simulink model "Bicycle_Model"  (R2019b)
settings: Solver=ode45  StartTime=0.0  StopTime=10.0  MaxStep=0.2  RelTol=1e-3
libraries: simulink x2
settings Model: Creator=Liam  LastModifiedBy=yafta
settings DataIOCC: ReturnWorkspaceOutputs=off
settings DebuggingCC: ArithmeticOperatorsInVariantConditions=warning
settings SFSimCC: SimUseLocalCustomCode=off  CustomCodeUndefinedFunction=UseInterfaceOnly
settings RTWCC: RTWUseLocalCustomCode=off

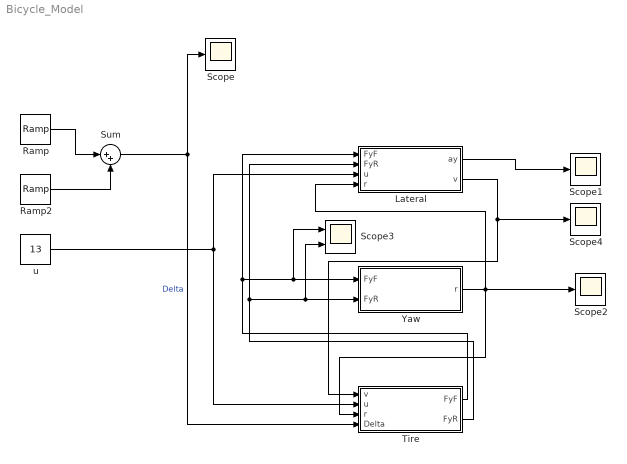
== system Bicycle_Model ==
  Lateral : Subsystem
  Ramp : simulink/Sources/Ramp  slope=0.05  start=1  InitialOutput=0
  Ramp2 : simulink/Sources/Ramp  slope=-0.05  start=5  InitialOutput=0
  Scope{,1..2,4} (4 alike) : Scope
  Scope3 : Scope  NumInputPorts=2
  Sum : Sum  Inputs=|++
  Tire : Subsystem
  Yaw : Subsystem
  u : Constant  Value=13
  wires:
  u/1 -> Tire/2(u), Lateral/3(u)
  Yaw/1(r) -> Lateral/4(r), Tire/3(r), Scope2/1
  Tire/1(FyF) -> Lateral/1(FyF), Scope3/1, Yaw/1("FyF ")
  Tire/2(FyR) -> Lateral/2(FyR), Scope3/2, Yaw/2(FyR)
  Ramp/1 -> Sum/1
  Ramp2/1 -> Sum/2
  Sum/1 -> Scope/1, Tire/4("Delta ")  "Delta"
  Lateral/1(ay) -> Scope1/1
  Lateral/2(v) -> Tire/1(v), Scope4/1

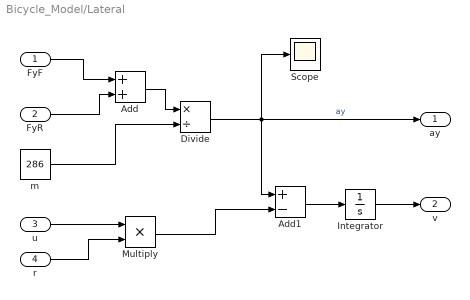
== system Bicycle_Model/Lateral ==
  FyF : Inport
  FyR : Inport  Port=2
  u : Inport  Port=3
  r : Inport  Port=4
  Add : Sum
  Add1 : Sum  Inputs=+-
  Divide : Product  Inputs=*/
  Integrator : Integrator
  Multiply : Product
  Scope : Scope
  m : Constant  Value=286
  ay : Outport  VectorParamsAs1DForOutWhenUnconnected=off
  v : Outport  Port=2  VectorParamsAs1DForOutWhenUnconnected=off
  wires:
  FyF/1 -> Add/1
  FyR/1 -> Add/2
  Add/1 -> Divide/1
  Divide/1 -> ay/1, Add1/1, Scope/1  "ay"
  m/1 -> Divide/2
  u/1 -> Multiply/1
  r/1 -> Multiply/2
  Multiply/1 -> Add1/2
  Add1/1 -> Integrator/1
  Integrator/1 -> v/1

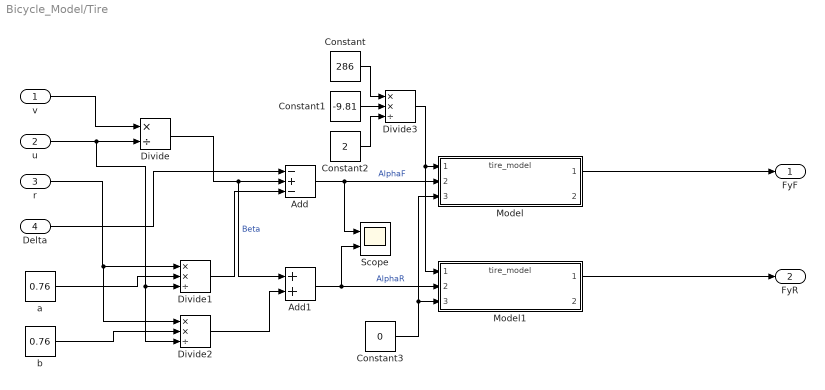
== system Bicycle_Model/Tire ==
  v : Inport
  u : Inport  Port=2
  r : Inport  Port=3
  "Delta " : Inport  Port=4
  Add : Sum  Inputs=-+-
  Add1 : Sum
  Constant : Constant  Value=286
  Constant1 : Constant  Value=-9.81
  Constant2 : Constant  Value=2
  Constant3 : Constant  Value=0
  Divide : Product  Inputs=*/
  Divide1 : Product  Inputs=**/
  Divide2 : Product  Inputs=**/
  Divide3 : Product  Inputs=**/
  Model : ModelReference  ModelNameDialog=tire_model.slx  SimulationMode=Normal  ModelReferenceVersion=1.6
  Model1 : ModelReference  ModelNameDialog=tire_model.slx  SimulationMode=Normal  ModelReferenceVersion=1.6
  Scope : Scope  NumInputPorts=2
  a : Constant  Value=0.76
  b : Constant  Value=0.76
  FyF : Outport  VectorParamsAs1DForOutWhenUnconnected=off
  FyR : Outport  Port=2  VectorParamsAs1DForOutWhenUnconnected=off
  wires:
  v/1 -> Divide/1
  u/1 -> Divide2/3, Divide1/3, Divide/2
  Divide/1 -> Add1/1, Add/2  "Beta"
  "Delta "/1 -> Add/1
  r/1 -> Divide2/1, Divide1/1
  a/1 -> Divide1/2
  Divide1/1 -> Add/3
  Add/1 -> Model/2, Scope/1  "AlphaF"
  b/1 -> Divide2/2
  Divide2/1 -> Add1/2
  Add1/1 -> Model1/2, Scope/2  "AlphaR"
  Model1/1 -> FyR/1
  Model/1 -> FyF/1
  Constant/1 -> Divide3/1
  Constant1/1 -> Divide3/2
  Constant2/1 -> Divide3/3
  Divide3/1 -> Model1/1, Model/1
  Constant3/1 -> Model1/3, Model/3

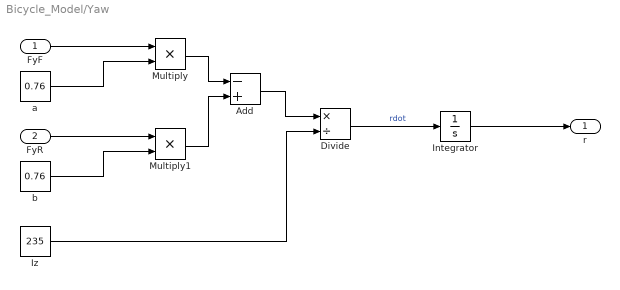
== system Bicycle_Model/Yaw ==
  "FyF " : Inport
  FyR : Inport  Port=2
  Add : Sum  Inputs=-+
  Divide : Product  Inputs=*/
  Integrator : Integrator
  Iz : Constant  Value=235
  Multiply : Product
  Multiply1 : Product
  a : Constant  Value=0.76
  b : Constant  Value=0.76
  r : Outport  VectorParamsAs1DForOutWhenUnconnected=off
  wires:
  "FyF "/1 -> Multiply/1
  a/1 -> Multiply/2
  FyR/1 -> Multiply1/1
  b/1 -> Multiply1/2
  Multiply/1 -> Add/1
  Multiply1/1 -> Add/2
  Add/1 -> Divide/1
  Iz/1 -> Divide/2
  Divide/1 -> Integrator/1  "rdot"
  Integrator/1 -> r/1
